simulink model "CruiseControl_AdHocTest"  (R2020a)
settings: configuration reference "ModelReferencingVisual" (kept outside this file)
settings Model: DataDictionary=CruiseControl_Req_dd.sldd  EnablePacing=on  Creator=yleong  LastModifiedBy=promero
settings ConfigSetRef: SourceName=ModelReferencingVisual

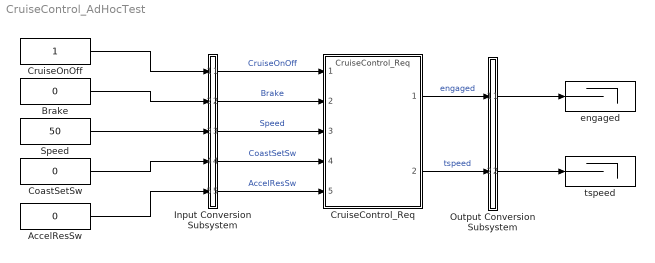
== system CruiseControl_AdHocTest ==
  AccelResSw : Constant  Value=0  OutDataTypeStr=boolean  SampleTime=0.1
  Brake : Constant  Value=0  OutDataTypeStr=boolean  SampleTime=0.1
  CoastSetSw : Constant  Value=0  OutDataTypeStr=boolean  SampleTime=0.1
  CruiseControl_Req : ModelReference  ModelNameDialog=CruiseControl_Req  SimulationMode=Normal  ModelReferenceVersion=1.468
  CruiseOnOff : Constant  OutDataTypeStr=boolean  SampleTime=0.1
  Input Conversion Subsystem : Subsystem  Tag=__SLT_ICS__  Description=|
      | Signal spec.
      | and routing
      settings: AttributesFormatString=%<Description>
  Output Conversion Subsystem : Subsystem  Tag=__SLT_OCS__  Description=|
      | Signal spec.
      | and routing
      settings: AttributesFormatString=%<Description>
  Speed : Constant  Value=50  OutDataTypeStr=uint8  SampleTime=0.1
  engaged : Terminator
  tspeed : Terminator
  wires:
  CruiseOnOff/1 -> Input Conversion Subsystem/1(Inport_1)
  Brake/1 -> Input Conversion Subsystem/2(Inport_2)
  Speed/1 -> Input Conversion Subsystem/3(Inport_3)
  CoastSetSw/1 -> Input Conversion Subsystem/4(Inport_4)
  AccelResSw/1 -> Input Conversion Subsystem/5(Inport_5)
  Output Conversion Subsystem/1(Outport_1) -> engaged/1
  Output Conversion Subsystem/2(Outport_2) -> tspeed/1
  Input Conversion Subsystem/1(Outport_1) -> CruiseControl_Req/1  "CruiseOnOff"
  Input Conversion Subsystem/2(Outport_2) -> CruiseControl_Req/2  "Brake"
  Input Conversion Subsystem/3(Outport_3) -> CruiseControl_Req/3  "Speed"
  Input Conversion Subsystem/4(Outport_4) -> CruiseControl_Req/4  "CoastSetSw"
  Input Conversion Subsystem/5(Outport_5) -> CruiseControl_Req/5  "AccelResSw"
  CruiseControl_Req/1 -> Output Conversion Subsystem/1(Inport_1)  "engaged"
  CruiseControl_Req/2 -> Output Conversion Subsystem/2(Inport_2)  "tspeed"

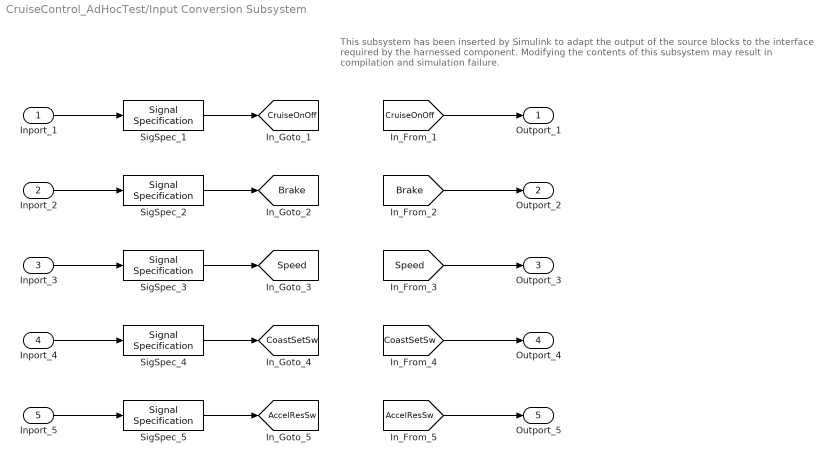
== system CruiseControl_AdHocTest/Input Conversion Subsystem ==
  note: This subsystem has been inserted by Simulink to adapt the output of the source blocks to the interface required by the harnessed component.
      |  Modifying the contents of this subsystem may result in compilation and simulation failure.
  Inport_1 : Inport
  Inport_2 : Inport  Port=2
  Inport_3 : Inport  Port=3
  Inport_4 : Inport  Port=4
  Inport_5 : Inport  Port=5
  SigSpec_{1..2,4..5} (4 alike) : SignalSpecification  OutDataTypeStr=boolean  Dimensions=[1]  SampleTime=0.1
  SigSpec_3 : SignalSpecification  OutDataTypeStr=uint8  Dimensions=[1]  SampleTime=0.1
  Outport_1 : Outport
  Outport_2 : Outport  Port=2
  Outport_3 : Outport  Port=3
  Outport_4 : Outport  Port=4
  Outport_5 : Outport  Port=5
  tag scope: AccelResSw=global, Brake=global, CoastSetSw=global, CruiseOnOff=global, Speed=global
  wires:
  [CruiseOnOff] -> Outport_1/1
  SigSpec_1/1 -> [CruiseOnOff]
  Inport_1/1 -> SigSpec_1/1
  [Brake] -> Outport_2/1
  SigSpec_2/1 -> [Brake]
  Inport_2/1 -> SigSpec_2/1
  [Speed] -> Outport_3/1
  SigSpec_3/1 -> [Speed]
  Inport_3/1 -> SigSpec_3/1
  [CoastSetSw] -> Outport_4/1
  SigSpec_4/1 -> [CoastSetSw]
  Inport_4/1 -> SigSpec_4/1
  [AccelResSw] -> Outport_5/1
  SigSpec_5/1 -> [AccelResSw]
  Inport_5/1 -> SigSpec_5/1

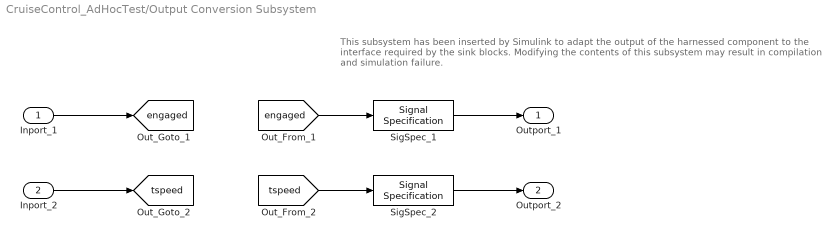
== system CruiseControl_AdHocTest/Output Conversion Subsystem ==
  note: This subsystem has been inserted by Simulink to adapt the output of the harnessed component to the interface required by the sink blocks.
      |  Modifying the contents of this subsystem may result in compilation and simulation failure.
  Inport_1 : Inport
  Inport_2 : Inport  Port=2
  SigSpec_1 : SignalSpecification  OutDataTypeStr=boolean  Dimensions=[1]  SampleTime=0.1
  SigSpec_2 : SignalSpecification  OutDataTypeStr=uint8  Dimensions=[1]  SampleTime=0.1
  Outport_1 : Outport
  Outport_2 : Outport  Port=2
  tag scope: engaged=global, tspeed=global
  wires:
  Inport_1/1 -> [engaged]
  [engaged] -> SigSpec_1/1
  SigSpec_1/1 -> Outport_1/1
  Inport_2/1 -> [tspeed]
  [tspeed] -> SigSpec_2/1
  SigSpec_2/1 -> Outport_2/1
